simulink model "TaskAllocation"  (R2015a)
settings: Solver=ode45  StartTime=0.0  StopTime=10.0  RelTol=1e-3
settings Model: Creator=ominub  LastModifiedBy=ominub

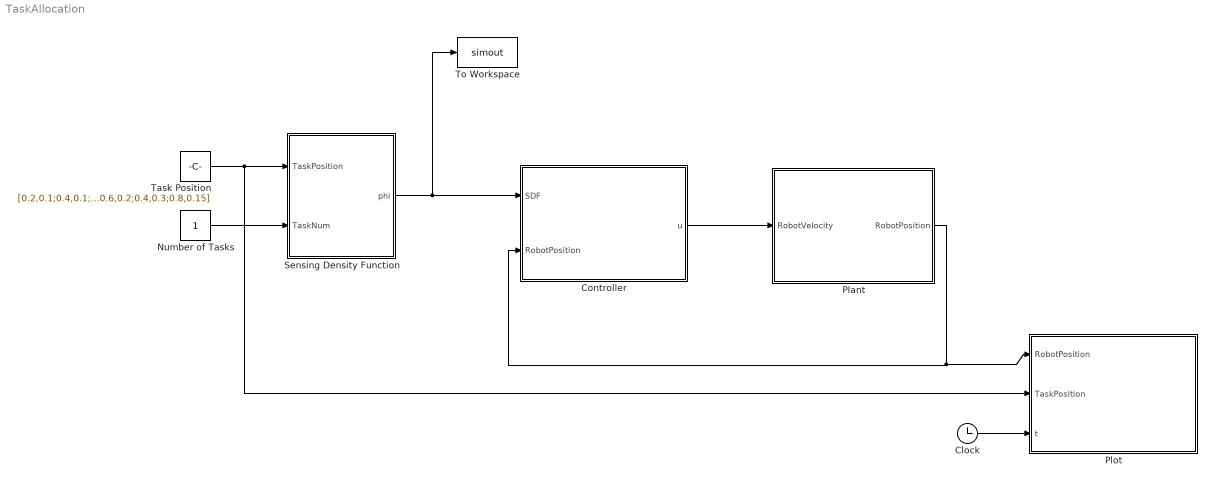
== system TaskAllocation ==
  Clock : Clock
  Controller : MATLAB Function  TreatAsAtomicUnit=on
  Number of Tasks : Constant
  Plant : Subsystem
  Plot : MATLAB Function  TreatAsAtomicUnit=on
  Sensing Density Function : MATLAB Function  TreatAsAtomicUnit=on
  Task Position : Constant  Value=[0.2,0.1;0.4,0.1;0.6,0.2;0.4,0.3;0.8,0.15]
  To Workspace : ToWorkspace  VariableName=simout  SaveFormat=Timeseries  SampleTime=-1
  wires:
  Number of Tasks/1 -> Sensing Density Function/2(TaskNum)
  Task Position/1 -> Plot/2(TaskPosition), Sensing Density Function/1(TaskPosition)
  Sensing Density Function/1(phi) -> To Workspace/1, Controller/1(SDF)
  Controller/1(u) -> Plant/1(RobotVelocity)
  Plant/1(RobotPosition) -> Controller/2(RobotPosition), Plot/1(RobotPosition)
  Clock/1 -> Plot/3(t)

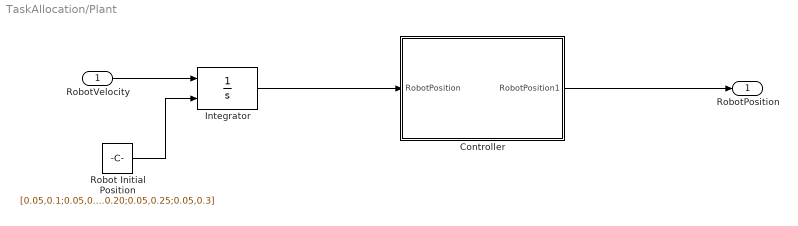
== system TaskAllocation/Plant ==
  RobotVelocity : Inport
  Controller : MATLAB Function  TreatAsAtomicUnit=on
  Integrator : Integrator  InitialConditionSource=external
  Robot Initial Position : Constant  Value=[0.05,0.1;0.05,0.15;0.05,0.20;0.05,0.25;0.05,0.3]
  RobotPosition : Outport
  wires:
  Robot Initial Position/1 -> Integrator/2
  RobotVelocity/1 -> Integrator/1
  Integrator/1 -> Controller/1(RobotPosition)
  Controller/1(RobotPosition1) -> RobotPosition/1

== matlab function TaskAllocation/Plant/Controller ==
  data: RobotPosition1 output; RobotPosition input
function RobotPosition1 = fcn(RobotPosition)
%avoid robots go out of environment  
%Actually, if robot go out of environment, it may implies the controller is
%unstable
RobotPosition1=ones(5,2);
    for m=1:1:length(RobotPosition(:,1))
        if RobotPosition(m,1)>1
            RobotPosition1(m,1)=1;
        elseif RobotPosition(m,1)<0
            RobotPosition1(m,1)=0;
        else
            RobotPosition1(m,1)=RobotPosition(m,1);
        end
        
        if RobotPosition(m,2)>0.4
            RobotPosition1(m,2)=0.4;
        elseif RobotPosition(m,2)<0
            RobotPosition1(m,2)=0;
        else
            RobotPosition1(m,2)=RobotPosition(m,2);
        end
    end
end

== matlab function TaskAllocation/Controller ==
  data: u output; SDF input; RobotPosition input
function u = fcn(SDF,RobotPosition)
% This block supports an embeddable subset of the MATLAB language.
% See the help menu for details.
x=0:0.01:1;
y=0:0.01:0.4;
u=zeros(length(RobotPosition(:,1)),2);
robotR=0.08;

    for i=1:1:length(SDF(:,1))
        for j=1:1:length(SDF(1,:))
            
            q=[x(i), y(j)];
          
            dphi=SDF(i,j);
            %Assumption of SDF
            if dphi<0
                dphi=0;
            end
            %penalty function
            d=1;
            for coverbot=1:1:length(RobotPosition(:,1))
                
                d=d-exp(-norm(q-RobotPosition(coverbot,:))^2/(2*robotR^2));
                
            end
%             [d,z]=max([0 d]);
             h=d^2;
             dh=2*d;
%              if z==1
%                     h=0;
%                     dh=0;
%              end
             
           
             
            for whichrobot=1:1:length(RobotPosition(:,1))
                u(whichrobot,:)= u(whichrobot,:)+(RobotPosition(whichrobot,:)-q)*dh*dphi*exp(-norm(q-RobotPosition(whichrobot,:))^2/(2*robotR^2));
                 
            end
        end
        
    end
    Km=1;
% Km=100;
    u=-Km*u;
end

== matlab function TaskAllocation/Plot ==
  data: RobotPosition input; TaskPosition input; t input
function  fcn(RobotPosition,TaskPosition,t)
% This block supports an embeddable subset of the MATLAB language.
% See the help menu for details.
x=0:0.01:1;
y=0:0.01:0.4;
 % plot
    figure('Position',[100 100 900 400])
%     subplot(2,1,1)
    plot(TaskPosition(:,1),TaskPosition(:,2),'^')
    hold on
    plot(RobotPosition(:,1),RobotPosition(:,2),'*')
    hold on
    %  for texti=1:1:length(EnvironData(:,1))
    %      for textj=1:1:length(EnvironData(1,:))
    %         t=num2str (EnvironData(texti,textj));
    %         text(x(texti)-0.45,y(textj)-0.45, t);
    %      end
    %  end
    
%     for num=1:1:length(SensorData(:,1))
%         t=num2str (SensorData(num));
%         text(SensorPosition(num,2)+0.05,SensorPosition(num,1)+0.05, t);
%     end
    axis([0 1 0 0.4])
%     voronoi(RobotPosition(:,1),RobotPosition(:,2))
    grid on
    

   
% %save files
%     picname=sprintf('%d.jpg',t);
%     saveas(gcf,picname);
end

== matlab function TaskAllocation/Sensing Density Function ==
  data: phi output; TaskPosition input; TaskNum input
function phi = fcn(TaskPosition,TaskNum)
% This block supports an embeddable subset of the MATLAB language.
% See the help menu for details.
x=0:0.01:1;
y=0:0.01:0.4;
phi=zeros(length(x),length(y));
taskR=0.02;
for i=1:1:length(x)
    for j=1:1:length(y)
        q=[x(i) y(j)];
        %Task
        for task=1:1:TaskNum
            if norm(q-TaskPosition(task,:))<2*taskR
              phi(i,j)=phi(i,j)+10*(exp(-norm(q-TaskPosition(task,:))^2/(2*taskR^2)));
            end
        end
        %Station
%         phi(i,j)=phi(i,j)+(TaskNumber-length(TaskPosition(:,1)))*10*(exp(-norm(q-StationPosition(1,:))^2/(2*0.02^2)));
    end
end
